simulink model "inverter"  (R2024b)
settings: Solver=VariableStepAuto  StartTime=0.0  StopTime=86400  RelTol=1e-3
libraries: spsSeriesRLCBranchLib x6, spsVariableResistorLib x4, spsVariableInductorLib x3, spsPVArrayLib x2, spsThreePhaseParallelRLCLoadLib x2, spsBoostConverterLib x1, spsParallelRLCBranchLib x1, spsGroundLib x1, spsTwoLevelConverterLib x1, spsPWMGeneratorDCDCLib x1, spsPWMGenerator2LevelLib x1, eePowerMeasurement x1
settings Model: Creator=DELL  LastModifiedBy=DELL

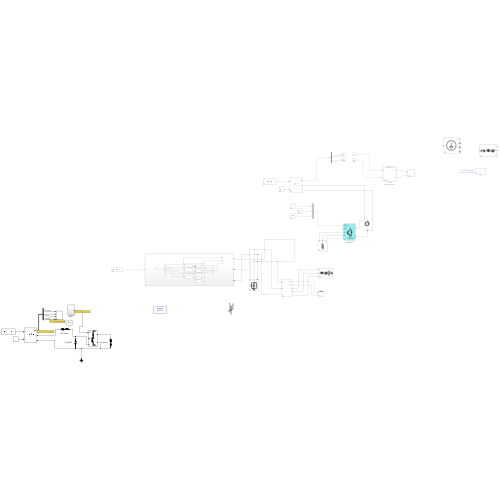
[thumbnail: Simulink's stored preview of the top-level diagram]
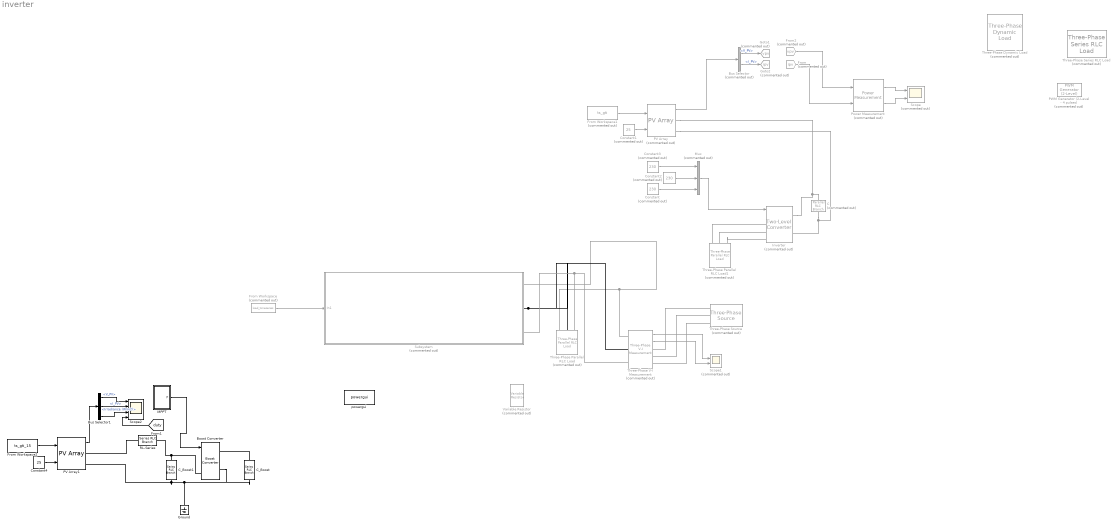
== system inverter ==
  Boost Converter : spsBoostConverterLib/Boost Converter  ModelType=Average model (D-controlled)  Ron=1e-3  Rs=1e6  Cs=inf  Vforward=[0,0]  Ron_Diode=1e-3  Rs_Diode=1e6  Cs_Diode=inf  Vf_Diode=1e-3  Rs_CurrentSource=inf  Ron_ACsource=1e-3
      settings: LibrarySourceBlock=sps_lib/Power Electronics/Boost Converter
  Bus Selector : BusSelector  Commented=on  OutputSignals=V_PV,I_PV
  Bus Selector1 : BusSelector  OutputSignals=V_PV,I_PV,Irradiance (W/m2)
  C : spsParallelRLCBranchLib/Parallel RLC Branch  Commented=on  LConnTagsString=a  RConnTagsString=__new0  BranchType=RC  Resistance=100  Inductance=inf  SetiL0=off  InitialCurrent=0  Capacitance=500e-06  Setx0=off  InitialVoltage=775  Measurements=Branch voltage
  C_Boost : spsSeriesRLCBranchLib/Series RLC Branch  LConnTagsString=__new0  RConnTagsString=__new0  BranchType=RC  Resistance=1e-5  Inductance=1e-3  SetiL0=off  InitialCurrent=0  Capacitance=100e-6  Setx0=off  InitialVoltage=230  Measurements=Branch voltage and current
  C_Boost1 : spsSeriesRLCBranchLib/Series RLC Branch  LConnTagsString=__new0  RConnTagsString=__new0  BranchType=C  Resistance=1e-5  Inductance=1e-3  SetiL0=off  InitialCurrent=0  Capacitance=10e-6  Setx0=off  InitialVoltage=230  Measurements=Branch voltage and current
  Constant : Constant  Commented=on  Value=230
  Constant1 : Constant  Commented=on  Value=25
  Constant2 : Constant  Commented=on  Value=230
  Constant3 : Constant  Commented=on  Value=230
  Constant4 : Constant  Value=25
  From : From  Commented=on  GotoTag=ipv  TagVisibility=global
  From Workspace : FromWorkspace  Commented=on  VariableName=load_timeseries  OutDataTypeStr=double  SampleTime=3600
  From Workspace1 : FromWorkspace  Commented=on  VariableName=ts_gti  OutDataTypeStr=double  SampleTime=3600
  From Workspace2 : FromWorkspace  VariableName=ts_gti_15  OutDataTypeStr=double
  From2 : From  Commented=on  GotoTag=vpv  TagVisibility=global
  Goto1 : Goto  Commented=on  GotoTag=vpv  TagVisibility=global
  Goto2 : Goto  Commented=on  GotoTag=ipv  TagVisibility=global
  Ground : spsGroundLib/Ground  LConnTagsString=a
  Inverter : spsTwoLevelConverterLib/Two-Level Converter  Commented=on  ModelType=Average model (No rectifier mode)  Ron=1e-3  Rs=1e6  Cs=inf  Vforward=[0,0]  Ron_Diode=1e-3  Rs_Diode=1e6  Cs_Diode=inf  Vf_Diode=1e-3  Rs_CurrentSource=inf  Ron_ACsource=1e-3
      settings: LibrarySourceBlock=sps_lib/Power Electronics/Two-Level Converter
  MPPT : Subsystem
  Mux : Mux  Commented=on  Inputs=3
  PV Array : spsPVArrayLib/PV Array  Commented=on  Npar=7  Nser=6  PlotType=array @ 1000 W/m2 & specified temperatures  S_vec="[ 1000  500  100 ]"  Temp_C_vec="[ 45 25  ]"  ModuleName=SunPower SPR-415E-WHT-D  PlotWhenSelected=off  Pm=414.801  Ncell=128  Voc=85.3  Isc=6.09  Vm=72.9  Im=5.69  beta_Voc_pc=-0.229  alpha_Isc_pc=0.030706  beta_Voc=-0.19534  alpha_Isc=0.00187  IL=6.0978  I0=7.1698e-13  nI=0.87223  Rsh=419.7781  Rs=0.53711  RobustModel=off  RobustCellTemperature=313.3991  BAL=on  Tc=1e-6  Tfilter=5e-5
  PV Array1 : spsPVArrayLib/PV Array  Npar=6  Nser=4  PlotType=array @ 1000 W/m2 & specified temperatures  S_vec="[ 1000  500  100 ]"  Temp_C_vec="[ 45 25  ]"  ModuleName=SunPower SPR-415E-WHT-D  PlotWhenSelected=off  Pm=414.801  Ncell=128  Voc=85.3  Isc=6.09  Vm=72.9  Im=5.69  beta_Voc_pc=-0.229  alpha_Isc_pc=0.030706  beta_Voc=-0.19534  alpha_Isc=0.00187  IL=6.0978  I0=7.1698e-13  nI=0.87223  Rsh=419.7781  Rs=0.53711  RobustModel=off  RobustCellTemperature=313.3991  BAL=on  Tc=1e-6  Tfilter=5e-5
  PWM Generator (2-Level - 4 pulses) : spsPWMGenerator2LevelLib/PWM Generator (2-Level)  Commented=on  ModulatorType=Three-phase bridge (6 pulses)  ModulatorMode=Unsynchronized  Fc=2000  Pc=90  nF=27  MinMax="[ -1  1 ]"  SamplingTechnique=Natural  ModulatingSignals=on  m=0.8  Freq=50  Phase=0  Ts=4e-6  ShowCarrierOutport=off
  Power Measurement : eePowerMeasurement/Power Measurement  Commented=on  LabelModeActiveChoice=Continuous  F=60  K=[0 1 2 3]  Ts=0
  RL-Series : spsSeriesRLCBranchLib/Series RLC Branch  LConnTagsString=__new0  RConnTagsString=__new0  BranchType=RL  Resistance=1e-3  Inductance=1e-3  SetiL0=off  InitialCurrent=0  Capacitance=100e-6  Setx0=off  InitialVoltage=230  Measurements=Branch voltage and current
  Scope : Scope  Commented=on  NumInputPorts=2
  Scope1 : Scope  Commented=on  NumInputPorts=2
  Scope2 : Scope  NumInputPorts=4
  Subsystem : Subsystem  Commented=on
  Three-Phase Dynamic Load : spsThreePhaseDynamicLoadLib/Three-Phase Dynamic Load  Commented=on  NominalVoltage=[ 500e3 60 ]  ActiveReactivePowers=[5e+007 2.5e+007]  PositiveSequence=[0.98441 -1.41063]  ExternalControl=on  NpNq=[1.3 2]  TimeConstants="[0  0  0  0]"  MinimumVoltage=0.7  Tfilter=1e-4  LoadFlowParameters=[4,0,0,0,0]
      settings: LibrarySourceBlock=|
      | sps_lib/Passives/Three-Phase
      | Dynamic Load
  Three-Phase Parallel RLC Load : spsThreePhaseParallelRLCLoadLib/Three-Phase Parallel RLC Load  Commented=on  LConnTagsString=A|B|C  Configuration=Y (grounded)  NominalVoltage=400  Vabc=[1e3 1e3 1e3]  Vabcp=[1e3 1e3 1e3]  NominalFrequency=60  UnbalancedPower=off  ActivePower=10e3  InductivePower=100  CapacitivePower=100  Pabc=[10e3 9e3 11e3]  QLabc=[100 90 110]  QCabc=[100 90 110]  Pabcp=[10e3 9e3 11e3]  QLabcp=[100 90 110]  QCabcp=[100 90 110]  Measurements=None  LoadType=constant Z
  Three-Phase Parallel RLC Load1 : spsThreePhaseParallelRLCLoadLib/Three-Phase Parallel RLC Load  Commented=on  LConnTagsString=A|B|C  Configuration=Delta  NominalVoltage=400  Vabc=[1e3 1e3 1e3]  Vabcp=[0.4e3 0.4e3 0.4e3]  NominalFrequency=60  UnbalancedPower=on  ActivePower=10e3  InductivePower=0  CapacitivePower=0  Pabc=[10e3 9e3 11e3]  QLabc=[100 90 110]  QCabc=[100 90 110]  Pabcp=[2e3 3e3 4e3]  QLabcp=[0 0 0]  QCabcp=[0 0 0]  Measurements=None  LoadType=constant Z
  Three-Phase Series RLC Load : spsThreePhaseSeriesRLCLoadLib/Three-Phase Series RLC Load  Commented=on  LConnTagsString=A|B|C  Configuration=Y (grounded)  NominalVoltage=1000  Vabc=[1e3 1e3 1e3]  Vabcp=[1e3 1e3 1e3]  NominalFrequency=60  UnbalancedPower=off  ActivePower=10e3  InductivePower=100  CapacitivePower=100  Pabc=[10e3 9e3 11e3]  QLabc=[100 90 110]  QCabc=[100 90 110]  Pabcp=[10e3 9e3 11e3]  QLabcp=[100 90 110]  QCabcp=[100 90 110]  Measurements=None  LoadType=constant Z
  Three-Phase V-I Measurement : spsThreePhaseVIMeasurementLib/Three-Phase V-I Measurement  Commented=on  VoltageMeasurement=phase-to-ground  SetLabelV=off  LabelV=Vabc  Vpu=off  VpuLL=off  CurrentMeasurement=yes  SetLabelI=off  LabelI=Iabc  Ipu=off  Pbase=100e6  Vbase=500e3  OutputType=Complex  PhasorSimulation=off  PSBequivalent=0
  Three-Phase Source : spsThreePhaseSourceLib/Three-Phase Source  Commented=on  InternalConnection=Yg  VoltagePhases=off  Voltage=400  PhaseAngle=0  Voltage_phases=[25e3 25e3 25e3]/sqrt(3)  PhaseAngles_phases=[0 -120 +120]  Frequency=60  NonIdealSource=on  SpecifyImpedance=off  Resistance=0.8929  Inductance=16.58e-3  ShortCircuitLevel=100e6  BaseVoltage=25e3  XRratio=7  BusType=swing  Pref=10e3  Qref=0  Prefabc=[10e3, 10e3, 10e3]  Qrefabc=[0, 0, 0]  Qmin=-inf  Qmax=inf
  Variable Resistor : spsVariableResistorLib/Variable Resistor  Commented=on  Rabsmin=100
      settings: LibrarySourceBlock=sps_lib/Passives/Variable Resistor
  powergui : spspowerguiLib/powergui  Priority=1  SimulationMode=Discrete  SampleTime=0.005  frequency=60  Iterations=50  frequencyindice=0  Pbase=100e6  ErrMax=1e-4  UnitsV=kV  UnitsW=MW  buscounter=0  FunctionMessages=off  echomessages=off  EnableUseOfTLC=off  CurrentSourceSwitches=off  DisableSnubberDevices=off  DisableRonSwitches=off  DisableVfSwitches=off  DisplayEquations=off  AutomaticDiscreteSolvers=off  SolverType=Tustin/Backward Euler (TBE)  Interpol=off  ExternalGateDelay=off  methode=off  Ts=100  x0status=blocks  SPID=on  SwTol=0  HookPort=off  NonlinearTolerance=1e-4  nMaxIteration=100  ContinueOnMaxIteration=off  RestoreLinks=warning  ResistiveCurrentMeasurement=off  Frange=[0:2:500]  Ylog=off  Xlog=on  ShowGrid=off  save=off  variable=ZData  structure=0  ZoomFFT=off  StartTime=0.0  cycles=1  DisplayStyle=1  fundamental=60  FreqAxis=off  MaxFrequency=1000  frequencyindicesteady=1  RmsSteady=1  display=off
  wires:
  Constant3/1 -> Mux/1
  Constant2/1 -> Mux/2
  Constant/1 -> Mux/3
  Mux/1 -> Inverter/1
  PV Array/1 -> Bus Selector/1
  From Workspace1/1 -> PV Array/1
  Constant1/1 -> PV Array/2
  Bus Selector/1 -> Goto1/1  "<V_PV>"
  Bus Selector/2 -> Goto2/1  "<I_PV>"
  From2/1 -> Power Measurement/1
  From/1 -> Power Measurement/2
  Power Measurement/1 -> Scope/1
  From Workspace/1 -> Subsystem/1(In1)
  Three-Phase V-I Measurement/1 -> Scope1/1
  Three-Phase V-I Measurement/2 -> Scope1/2
  Power Measurement/2 -> Scope/2
  Constant4/1 -> PV Array1/2
  MPPT/1(P) -> Boost Converter/1
  From Workspace2/1 -> PV Array1/1
  PV Array1/1 -> Bus Selector1/1
  Bus Selector1/1 -> Scope2/1  "<V_PV>"
  Bus Selector1/2 -> Scope2/2  "<I_PV>"
  Bus Selector1/3 -> Scope2/3  "<Irradiance (W/m2)>"
  [duty] -> Scope2/4
  connections:
  C/RConn1 -- Inverter/RConn2 -- PV Array/RConn2
  Inverter/RConn1 -- PV Array/RConn1 -- C/LConn1
  Three-Phase Parallel RLC Load/LConn1 -- Subsystem/RConn1 -- Three-Phase V-I Measurement/LConn1
  Subsystem/RConn2 -- Three-Phase V-I Measurement/LConn2 -- Three-Phase Parallel RLC Load/LConn2
  Three-Phase Parallel RLC Load/LConn3 -- Three-Phase V-I Measurement/LConn3 -- Subsystem/RConn3
  Three-Phase Source/RConn1 -- Three-Phase V-I Measurement/RConn1
  Three-Phase Source/RConn2 -- Three-Phase V-I Measurement/RConn2
  Three-Phase Source/RConn3 -- Three-Phase V-I Measurement/RConn3
  Three-Phase Parallel RLC Load1/LConn1 -- Inverter/LConn1
  Three-Phase Parallel RLC Load1/LConn2 -- Inverter/LConn2
  Three-Phase Parallel RLC Load1/LConn3 -- Inverter/LConn3
  Ground/LConn1 -- C_Boost/RConn1 -- Boost Converter/RConn2 -- C_Boost1/RConn1 -- PV Array1/RConn2
  C_Boost/LConn1 -- Boost Converter/RConn1
  Boost Converter/LConn1 -- C_Boost1/LConn1 -- RL-Series/RConn1
  RL-Series/LConn1 -- PV Array1/RConn1

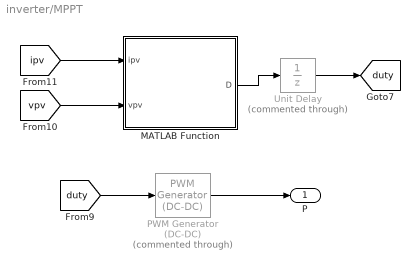
== system inverter/MPPT ==
  MATLAB Function : MATLAB Function  TreatAsAtomicUnit=on
  PWM Generator (DC-DC) : spsPWMGeneratorDCDCLib/PWM Generator (DC-DC)  Commented=through  Fsw=1000  Ts=0
  Unit Delay : UnitDelay  Commented=through  SampleTime=-1  HasFrameUpgradeWarning=on
  P : Outport
  tag scope: duty=global
  wires:
  [duty] -> PWM Generator (DC-DC)/1
  MATLAB Function/1(D) -> Unit Delay/1
  PWM Generator (DC-DC)/1 -> P/1
  [ipv] -> MATLAB Function/1(ipv)
  [vpv] -> MATLAB Function/2(vpv)
  Unit Delay/1 -> [duty]

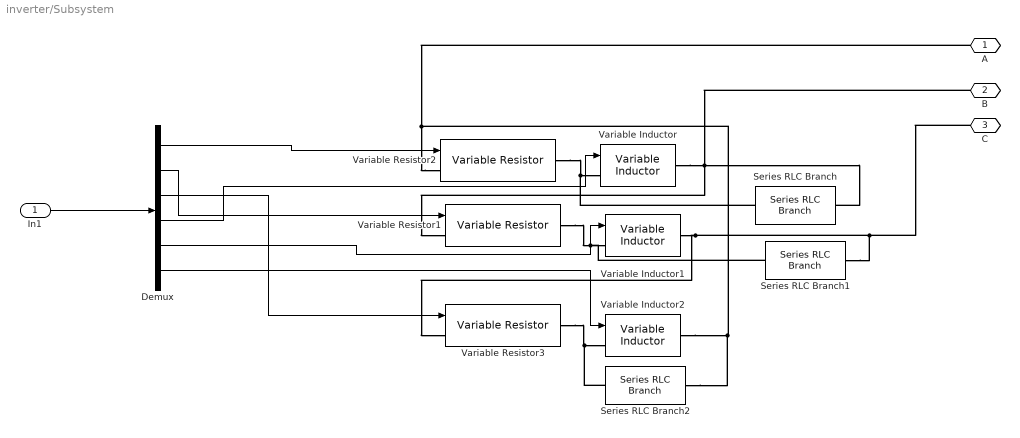
== system inverter/Subsystem ==
  In1 : Inport
  Demux : Demux  Outputs=6
  Series RLC Branch : spsSeriesRLCBranchLib/Series RLC Branch  LConnTagsString=__new0  RConnTagsString=__new0  BranchType=R  Resistance=1e3  Inductance=0  SetiL0=off  InitialCurrent=0  Capacitance=0  Setx0=off  InitialVoltage=0  Measurements=None
  Series RLC Branch1 : spsSeriesRLCBranchLib/Series RLC Branch  LConnTagsString=__new0  RConnTagsString=__new0  BranchType=R  Resistance=1e3  Inductance=0  SetiL0=off  InitialCurrent=0  Capacitance=0  Setx0=off  InitialVoltage=0  Measurements=None
  Series RLC Branch2 : spsSeriesRLCBranchLib/Series RLC Branch  LConnTagsString=__new0  RConnTagsString=__new0  BranchType=R  Resistance=1e3  Inductance=0  SetiL0=off  InitialCurrent=0  Capacitance=0  Setx0=off  InitialVoltage=0  Measurements=None
  Variable Inductor : spsVariableInductorLib/Variable Inductor  methode=Backward Euler  Labsmin=1e-6  Initialize=off  iL0=0  L0=1e-3  Vl0=0
      settings: LibrarySourceBlock=sps_lib/Passives/Variable Inductor
  Variable Inductor1 : spsVariableInductorLib/Variable Inductor  methode=Backward Euler  Labsmin=1e-6  Initialize=off  iL0=0  L0=1e-3  Vl0=0
      settings: LibrarySourceBlock=sps_lib/Passives/Variable Inductor
  Variable Inductor2 : spsVariableInductorLib/Variable Inductor  methode=Backward Euler  Labsmin=1e-6  Initialize=off  iL0=0  L0=1e-3  Vl0=0
      settings: LibrarySourceBlock=sps_lib/Passives/Variable Inductor
  Variable Resistor1 : spsVariableResistorLib/Variable Resistor  Rabsmin=1e-3
      settings: LibrarySourceBlock=sps_lib/Passives/Variable Resistor
  Variable Resistor2 : spsVariableResistorLib/Variable Resistor  Rabsmin=1e-3
      settings: LibrarySourceBlock=sps_lib/Passives/Variable Resistor
  Variable Resistor3 : spsVariableResistorLib/Variable Resistor  Rabsmin=1e-3
      settings: LibrarySourceBlock=sps_lib/Passives/Variable Resistor
  "A " : PMIOPort  Side=Right
  " B" : PMIOPort  Port=2  Side=Right
  " C" : PMIOPort  Port=3  Side=Right
  wires:
  Demux/2 -> Variable Resistor1/1
  Demux/5 -> Variable Inductor1/1
  Demux/3 -> Variable Resistor3/1
  Demux/1 -> Variable Resistor2/1
  Demux/4 -> Variable Inductor/1
  Demux/6 -> Variable Inductor2/1
  In1/1 -> Demux/1
  connections:
  Variable Resistor1/RConn1 -- Series RLC Branch1/LConn1 -- Variable Inductor1/LConn1
  Variable Inductor1/RConn1 -- " C"/RConn1 -- Series RLC Branch1/RConn1 -- Variable Resistor3/LConn1
  Variable Resistor3/RConn1 -- Series RLC Branch2/LConn1 -- Variable Inductor2/LConn1
  Variable Resistor2/LConn1 -- "A "/RConn1 -- Series RLC Branch2/RConn1 -- Variable Inductor2/RConn1
  Variable Inductor/RConn1 -- " B"/RConn1 -- Series RLC Branch/RConn1 -- Variable Resistor1/LConn1
  Variable Resistor2/RConn1 -- Series RLC Branch/LConn1 -- Variable Inductor/LConn1

== matlab function inverter/MPPT/MATLAB Function ==
  data: ipv input; D output; vpv input
function D = inccond_mppt(ipv, vpv)
    % Incremental Conductance MPPT algorithm for PV system (optimized for buck converter)
    % Inputs: ipv - PV current (A), vpv - PV voltage (V)
    % Output: D - Duty cycle (0.2 to 0.9)

    persistent I_prev V_prev D_prev;
    if isempty(I_prev)
        I_prev = 0;
        V_prev = 291; % Initial PV voltage (adjust based on PV array specs)
        D_prev = 0.5; % Initial duty cycle
    end

    delta_D = 0.005; % Step size for duty cycle adjustment
    D_min = 0.2;     % Minimum duty cycle
    D_max = 0.9;     % Maximum duty cycle
    tol = 1e-4;      % Tolerance for MPP detection
    v_min = 1e-3;    % Minimum voltage threshold

    % Check for invalid inputs
    if isnan(ipv) || isnan(vpv) || ipv < 0 || vpv < v_min
        D = D_prev;
        return;
    end

    % Calculate incremental changes
    delta_I = ipv - I_prev;
    delta_V = vpv - V_prev;

    % Handle small delta_V
    if abs(delta_V) < 1e-4
        if delta_I > 1e-4
            D = D_prev + delta_D; % Increase voltage (increase D for buck)
        elseif delta_I < -1e-4
            D = D_prev - delta_D; % Decrease voltage (decrease D)
        else
            D = D_prev; % No change
        end
    else
        % Calculate instantaneous and incremental conductance
        inst_cond = ipv / vpv; % I/V
        inc_cond = delta_I / delta_V; % dI/dV

        % Compare incremental and instantaneous conductance
        if abs(inc_cond + inst_cond) < tol
            D = D_prev; % At MPP
        elseif inc_cond > -inst_cond
            D = D_prev + delta_D; % Left of MPP, increase voltage (increase D)
        else
            D = D_prev - delta_D; % Right of MPP, decrease voltage (decrease D)
        end
    end

    % Limit duty cycle
    D = min(D_max, max(D_min, D));

    % Update previous values
    I_prev = ipv;
    V_prev = vpv;
    D_prev = D;
end
